simulink model "TorqueVect"  (R2022a)
settings: Solver=VariableStepAuto  StartTime=0.0  StopTime=300  RelTol=1e-3
PreLoadFcn:
  | run('Parameters\FSE_Parameters.m')
values from neighbouring files (symbols this model uses):
  Kd = 0;')    [open_carmaker_gui.m]
  Ki = 0    [open_carmaker_gui.m]
undefined symbols (not defined in the file or in its folder): BRegenEnabledButton, canChannel, CyalphaLookUp, efficiency, Fz_curve, Fz_scaling_long, gearR, izz, jw, kd, ki, Kp, kp, l_f, l_r, lambda, m, Mz_max, N, N_lat, N_long, P_max, pid_kd_lat, pid_kd_long, pid_ki_lat, pid_ki_long, pid_kp_lat, pid_kp_long, R_max, rw, steerR, T_i_max, TC_Decr_Gas, TC_Derivative, TC_Incr_Gas, TC_On, TC_Relay_Off, TC_Relay_On, tireCornerStiffness, Ts, TV_On, TV_Override, velocity_lookup, velocity_lookup_lat, y_ref, yrr_scaling
libraries: simulink x218, slpidlib x135, CarMaker4SL x73, TractionControlLibrary x13, canmsglib x9, canlib x8, TorqueVectoringLibrary x6, simulink_extras x4, PedalConversionLibrary x3, PowerControlLibrary x1
(part 9 of 26)

== system TorqueVect/CarMaker/IPG Vehicle/PowerTrain/PTControl Example/PTControl_ALL_Speedgoat/New TC/Reference Generator1 ==
  note: Modified slip ratio targets
  note: Vehicle velocity
  note: For throttle sign and Product:
      | If positive, normal reference
      | If negative (regen), similar reference but negative (negative target slip*times speed), this might need to change to account for regen limits
      | If 0, target zero
  x2 : Inport
  Front SR Target : Inport  Port=2
  Rear SR Target : Inport  Port=3
  Constant : Constant
  Product1 : Product
  Product2 : Product
  Switch : Switch  Criteria=u2 > Threshold  Threshold=1  SaturateOnIntegerOverflow=off  InputSameDT=off
  R1 : Outport
  L1 : Outport  Port=2
  R2 : Outport  Port=3
  L2 : Outport  Port=4
  wires:
  Front SR Target/1 -> Product1/1
  Product1/1 -> L1/1, R1/1
  Product2/1 -> L2/1, R2/1
  Rear SR Target/1 -> Product2/2
  Switch/1 -> Product2/1, Product1/2
  x2/1 -> Switch/1, Switch/2
  Constant/1 -> Switch/3

== system TorqueVect/CarMaker/IPG Vehicle/PowerTrain/PTControl Example/PTControl_ALL_Speedgoat/New TC/TC R1 ==
  modified slip ratio reference : Inport
  lim 1 : Inport  Port=2
  modified slip ratio measurement : Inport  Port=3
  P_TC : Inport  Port=4
  D_TC : Inport  Port=5
  enable_tc : Inport  Port=6
  PID Controller : slpidlib/PID Controller  Commented=on  Controller=PD  Form=Parallel  TimeDomain=Discrete-time  UseExternalTs=off  SampleTime=-1  IntegratorMethod=Forward Euler  FilterMethod=Forward Euler  ControllerParametersSource=external  P=125  I=1  UseKiTs=on  D=0  N=100  UseFilter=on  TunerSelectOption=Transfer Function Based (PID Tuner App)  InitialConditionSource=internal  InitialConditionForIntegrator=0  InitialConditionForFilter=0  DifferentiatorICPrevScaledInput=0  ExternalReset=none  TrackingMode=off  Kt=1  LimitOutput=on  SatLimitsSource=external  UpperSaturationLimit=inf  LowerSaturationLimit=-inf  LinearizeAsGain=on  AntiWindupMode=clamping  Kb=1  POutMin=[]  POutMax=[]  IOutMin=[]  IOutMax=[]  DOutMin=[]  DOutMax=[]  NOutMin=[]  NOutMax=[]  SumOutMin=[]  SumOutMax=[]  SaturationOutMin=[]  SaturationOutMax=[]  PParamMin=[]  PParamMax=[]  IParamMin=[]  IParamMax=[]  DParamMin=[]  DParamMax=[]  NParamMin=[]  NParamMax=[]  KbParamMin=[]  KbParamMax=[]  KtParamMin=[]  KtParamMax=[]  KbOutMin=[]  KbOutMax=[]  KtOutMin=[]  KtOutMax=[]  IntegratorOutMin=[]  IntegratorOutMax=[]  FilterOutMin=[]  FilterOutMax=[]  SumI1OutMin=[]  SumI1OutMax=[]  SumI2OutMin=[]  SumI2OutMax=[]  SumI3OutMin=[]  SumI3OutMax=[]  SumI4OutMin=[]  SumI4OutMax=[]  SumDOutMin=[]  SumDOutMax=[]  DifferentiatorOutMin=[]  DifferentiatorOutMax=[]  FilterDiffOutCoefMin=[]  FilterDiffOutCoefMax=[]  ReciprocalOutMin=[]  ReciprocalOutMax=[]  SumDenOutMin=[]  SumDenOutMax=[]  SumNumOutMin=[]  SumNumOutMax=[]  DivideOutMin=[]  DivideOutMax=[]  UdiffTsProdOutMin=[]  UdiffTsProdOutMax=[]  NTsProdOutMin=[]  NTsProdOutMax=[]  UintegralTsProdOutMin=[]  UintegralTsProdOutMax=[]  UngainTsProdOutMin=[]  UngainTsProdOutMax=[]  ClampingZeroOutDataTypeStr=Inherit: Inherit via back propagation  ClampingZeroOutMin=[]  ClampingZeroOutMax=[]  FilterDenConstantOutDataTypeStr=Inherit: Inherit via back propagation  FilterDenConstantOutMin=[]  FilterDenConstantOutMax=[]  PCopyOutDataTypeStr=Inherit: Inherit via back propagation  PCopyOutMin=[]  PCopyOutMax=[]  NCopyOutDataTypeStr=Inherit: Inherit via back propagation  NCopyOutMin=[]  NCopyOutMax=[]  IntegratorContinuousStateAttributes=''  IntegratorStateMustResolveToSignalObject=off  IntegratorRTWStateStorageClass=Auto  FilterContinuousStateAttributes=''  FilterStateMustResolveToSignalObject=off  FilterRTWStateStorageClass=Auto  ParallelPVariant=ExternalParameters  IdealPVariant=Disabled  IVariant=Disabled  DVariant=ExternalParameters  IntegratorVariant=Disabled  SatVariant=External  AWVariant=Disabled  PCopyVariant=Disabled  TRVariant=Disabled  FdbkBlocksVariant=Forward  IdealPFdbkVariant=Disabled  SatFdbkVariant=Disabled  DerivativeFilterVariant=ForwardEulerFilter  NVariant=ExternalParameters  NCopyVariant=Disabled  FilterICVariant=InternalICsFilter  IntegratorICVariant=Disabled  ExternalResetVariant=Disabled  TRSumVariant=Passthrough  SumFdbkVariant=Disabled  SumVariant=Sum_PD  TsampFilterVariant=InternalTs  TsampNgainVariant=Passthrough  TsampIntegralVariant=Disabled_SignalSpec  ExternalSaturationOutDataTypeStr=Inherit: Same as second input  aMode=0
  Sum1 : Sum  Inputs=|-+
  Sum2 : Sum  Commented=on  Inputs=|-+
  traction_controller : Subsystem
  Control Effort 1 : Outport
  wires:
  modified slip ratio reference/1 -> Sum1/1
  modified slip ratio measurement/1 -> Sum1/2
  lim 1/1 -> Sum2/2, traction_controller/1(max_torque)
  PID Controller/1 -> Sum2/1
  traction_controller/1(delta_torque) -> Control Effort 1/1
  enable_tc/1 -> traction_controller/3(enable_tc)
  Sum1/1 -> traction_controller/2(dslip)
  P_TC/1 -> traction_controller/4(Kp)
  D_TC/1 -> traction_controller/5(Kd)

== system TorqueVect/CarMaker/IPG Vehicle/PowerTrain/PTControl Example/PTControl_ALL_Speedgoat/New TC/TC R2 ==
  modified slip ratio reference : Inport
  lim 1 : Inport  Port=2
  modified slip ratio measurement : Inport  Port=3
  P_TC : Inport  Port=4
  D_TC : Inport  Port=5
  enable_tc : Inport  Port=6
  PID Controller : slpidlib/PID Controller  Commented=on  Controller=PD  Form=Parallel  TimeDomain=Discrete-time  UseExternalTs=off  SampleTime=-1  IntegratorMethod=Forward Euler  FilterMethod=Forward Euler  ControllerParametersSource=external  P=125  I=1  UseKiTs=on  D=0  N=100  UseFilter=on  TunerSelectOption=Transfer Function Based (PID Tuner App)  InitialConditionSource=internal  InitialConditionForIntegrator=0  InitialConditionForFilter=0  DifferentiatorICPrevScaledInput=0  ExternalReset=none  TrackingMode=off  Kt=1  LimitOutput=on  SatLimitsSource=external  UpperSaturationLimit=inf  LowerSaturationLimit=-inf  LinearizeAsGain=on  AntiWindupMode=clamping  Kb=1  POutMin=[]  POutMax=[]  IOutMin=[]  IOutMax=[]  DOutMin=[]  DOutMax=[]  NOutMin=[]  NOutMax=[]  SumOutMin=[]  SumOutMax=[]  SaturationOutMin=[]  SaturationOutMax=[]  PParamMin=[]  PParamMax=[]  IParamMin=[]  IParamMax=[]  DParamMin=[]  DParamMax=[]  NParamMin=[]  NParamMax=[]  KbParamMin=[]  KbParamMax=[]  KtParamMin=[]  KtParamMax=[]  KbOutMin=[]  KbOutMax=[]  KtOutMin=[]  KtOutMax=[]  IntegratorOutMin=[]  IntegratorOutMax=[]  FilterOutMin=[]  FilterOutMax=[]  SumI1OutMin=[]  SumI1OutMax=[]  SumI2OutMin=[]  SumI2OutMax=[]  SumI3OutMin=[]  SumI3OutMax=[]  SumI4OutMin=[]  SumI4OutMax=[]  SumDOutMin=[]  SumDOutMax=[]  DifferentiatorOutMin=[]  DifferentiatorOutMax=[]  FilterDiffOutCoefMin=[]  FilterDiffOutCoefMax=[]  ReciprocalOutMin=[]  ReciprocalOutMax=[]  SumDenOutMin=[]  SumDenOutMax=[]  SumNumOutMin=[]  SumNumOutMax=[]  DivideOutMin=[]  DivideOutMax=[]  UdiffTsProdOutMin=[]  UdiffTsProdOutMax=[]  NTsProdOutMin=[]  NTsProdOutMax=[]  UintegralTsProdOutMin=[]  UintegralTsProdOutMax=[]  UngainTsProdOutMin=[]  UngainTsProdOutMax=[]  ClampingZeroOutDataTypeStr=Inherit: Inherit via back propagation  ClampingZeroOutMin=[]  ClampingZeroOutMax=[]  FilterDenConstantOutDataTypeStr=Inherit: Inherit via back propagation  FilterDenConstantOutMin=[]  FilterDenConstantOutMax=[]  PCopyOutDataTypeStr=Inherit: Inherit via back propagation  PCopyOutMin=[]  PCopyOutMax=[]  NCopyOutDataTypeStr=Inherit: Inherit via back propagation  NCopyOutMin=[]  NCopyOutMax=[]  IntegratorContinuousStateAttributes=''  IntegratorStateMustResolveToSignalObject=off  IntegratorRTWStateStorageClass=Auto  FilterContinuousStateAttributes=''  FilterStateMustResolveToSignalObject=off  FilterRTWStateStorageClass=Auto  ParallelPVariant=ExternalParameters  IdealPVariant=Disabled  IVariant=Disabled  DVariant=ExternalParameters  IntegratorVariant=Disabled  SatVariant=External  AWVariant=Disabled  PCopyVariant=Disabled  TRVariant=Disabled  FdbkBlocksVariant=Forward  IdealPFdbkVariant=Disabled  SatFdbkVariant=Disabled  DerivativeFilterVariant=ForwardEulerFilter  NVariant=ExternalParameters  NCopyVariant=Disabled  FilterICVariant=InternalICsFilter  IntegratorICVariant=Disabled  ExternalResetVariant=Disabled  TRSumVariant=Passthrough  SumFdbkVariant=Disabled  SumVariant=Sum_PD  TsampFilterVariant=InternalTs  TsampNgainVariant=Passthrough  TsampIntegralVariant=Disabled_SignalSpec  ExternalSaturationOutDataTypeStr=Inherit: Same as second input  aMode=0
  Sum1 : Sum  Inputs=|-+
  Sum2 : Sum  Commented=on  Inputs=|-+
  traction_controller : Subsystem
  Control Effort 1 : Outport
  wires:
  modified slip ratio reference/1 -> Sum1/1
  modified slip ratio measurement/1 -> Sum1/2
  lim 1/1 -> Sum2/2, traction_controller/1(max_torque)
  PID Controller/1 -> Sum2/1
  traction_controller/1(delta_torque) -> Control Effort 1/1
  enable_tc/1 -> traction_controller/3(enable_tc)
  Sum1/1 -> traction_controller/2(dslip)
  P_TC/1 -> traction_controller/4(Kp)
  D_TC/1 -> traction_controller/5(Kd)

== system TorqueVect/CarMaker/IPG Vehicle/PowerTrain/PTControl Example/PTControl_ALL_Speedgoat/New TC/TC R3 ==
  modified slip ratio reference : Inport
  lim 1 : Inport  Port=2
  modified slip ratio measurement : Inport  Port=3
  P_TC : Inport  Port=4
  D_TC : Inport  Port=5
  enable_tc : Inport  Port=6
  PID Controller : slpidlib/PID Controller  Commented=on  Controller=PD  Form=Parallel  TimeDomain=Discrete-time  UseExternalTs=off  SampleTime=-1  IntegratorMethod=Forward Euler  FilterMethod=Forward Euler  ControllerParametersSource=external  P=125  I=1  UseKiTs=on  D=0  N=100  UseFilter=on  TunerSelectOption=Transfer Function Based (PID Tuner App)  InitialConditionSource=internal  InitialConditionForIntegrator=0  InitialConditionForFilter=0  DifferentiatorICPrevScaledInput=0  ExternalReset=none  TrackingMode=off  Kt=1  LimitOutput=on  SatLimitsSource=external  UpperSaturationLimit=inf  LowerSaturationLimit=-inf  LinearizeAsGain=on  AntiWindupMode=clamping  Kb=1  POutMin=[]  POutMax=[]  IOutMin=[]  IOutMax=[]  DOutMin=[]  DOutMax=[]  NOutMin=[]  NOutMax=[]  SumOutMin=[]  SumOutMax=[]  SaturationOutMin=[]  SaturationOutMax=[]  PParamMin=[]  PParamMax=[]  IParamMin=[]  IParamMax=[]  DParamMin=[]  DParamMax=[]  NParamMin=[]  NParamMax=[]  KbParamMin=[]  KbParamMax=[]  KtParamMin=[]  KtParamMax=[]  KbOutMin=[]  KbOutMax=[]  KtOutMin=[]  KtOutMax=[]  IntegratorOutMin=[]  IntegratorOutMax=[]  FilterOutMin=[]  FilterOutMax=[]  SumI1OutMin=[]  SumI1OutMax=[]  SumI2OutMin=[]  SumI2OutMax=[]  SumI3OutMin=[]  SumI3OutMax=[]  SumI4OutMin=[]  SumI4OutMax=[]  SumDOutMin=[]  SumDOutMax=[]  DifferentiatorOutMin=[]  DifferentiatorOutMax=[]  FilterDiffOutCoefMin=[]  FilterDiffOutCoefMax=[]  ReciprocalOutMin=[]  ReciprocalOutMax=[]  SumDenOutMin=[]  SumDenOutMax=[]  SumNumOutMin=[]  SumNumOutMax=[]  DivideOutMin=[]  DivideOutMax=[]  UdiffTsProdOutMin=[]  UdiffTsProdOutMax=[]  NTsProdOutMin=[]  NTsProdOutMax=[]  UintegralTsProdOutMin=[]  UintegralTsProdOutMax=[]  UngainTsProdOutMin=[]  UngainTsProdOutMax=[]  ClampingZeroOutDataTypeStr=Inherit: Inherit via back propagation  ClampingZeroOutMin=[]  ClampingZeroOutMax=[]  FilterDenConstantOutDataTypeStr=Inherit: Inherit via back propagation  FilterDenConstantOutMin=[]  FilterDenConstantOutMax=[]  PCopyOutDataTypeStr=Inherit: Inherit via back propagation  PCopyOutMin=[]  PCopyOutMax=[]  NCopyOutDataTypeStr=Inherit: Inherit via back propagation  NCopyOutMin=[]  NCopyOutMax=[]  IntegratorContinuousStateAttributes=''  IntegratorStateMustResolveToSignalObject=off  IntegratorRTWStateStorageClass=Auto  FilterContinuousStateAttributes=''  FilterStateMustResolveToSignalObject=off  FilterRTWStateStorageClass=Auto  ParallelPVariant=ExternalParameters  IdealPVariant=Disabled  IVariant=Disabled  DVariant=ExternalParameters  IntegratorVariant=Disabled  SatVariant=External  AWVariant=Disabled  PCopyVariant=Disabled  TRVariant=Disabled  FdbkBlocksVariant=Forward  IdealPFdbkVariant=Disabled  SatFdbkVariant=Disabled  DerivativeFilterVariant=ForwardEulerFilter  NVariant=ExternalParameters  NCopyVariant=Disabled  FilterICVariant=InternalICsFilter  IntegratorICVariant=Disabled  ExternalResetVariant=Disabled  TRSumVariant=Passthrough  SumFdbkVariant=Disabled  SumVariant=Sum_PD  TsampFilterVariant=InternalTs  TsampNgainVariant=Passthrough  TsampIntegralVariant=Disabled_SignalSpec  ExternalSaturationOutDataTypeStr=Inherit: Same as second input  aMode=0
  Sum1 : Sum  Inputs=|-+
  Sum2 : Sum  Commented=on  Inputs=|-+
  traction_controller : Subsystem
  Control Effort 1 : Outport
  wires:
  modified slip ratio reference/1 -> Sum1/1
  modified slip ratio measurement/1 -> Sum1/2
  lim 1/1 -> Sum2/2, traction_controller/1(max_torque)
  PID Controller/1 -> Sum2/1
  traction_controller/1(delta_torque) -> Control Effort 1/1
  enable_tc/1 -> traction_controller/3(enable_tc)
  Sum1/1 -> traction_controller/2(dslip)
  P_TC/1 -> traction_controller/4(Kp)
  D_TC/1 -> traction_controller/5(Kd)

== system TorqueVect/CarMaker/IPG Vehicle/PowerTrain/PTControl Example/PTControl_ALL_Speedgoat/New TC/TC R4 ==
  modified slip ratio reference : Inport
  lim 1 : Inport  Port=2
  modified slip ratio measurement : Inport  Port=3
  P_TC : Inport  Port=4
  D_TC : Inport  Port=5
  enable_tc : Inport  Port=6
  PID Controller : slpidlib/PID Controller  Commented=on  Controller=PD  Form=Parallel  TimeDomain=Discrete-time  UseExternalTs=off  SampleTime=-1  IntegratorMethod=Forward Euler  FilterMethod=Forward Euler  ControllerParametersSource=external  P=125  I=1  UseKiTs=on  D=0  N=100  UseFilter=on  TunerSelectOption=Transfer Function Based (PID Tuner App)  InitialConditionSource=internal  InitialConditionForIntegrator=0  InitialConditionForFilter=0  DifferentiatorICPrevScaledInput=0  ExternalReset=none  TrackingMode=off  Kt=1  LimitOutput=on  SatLimitsSource=external  UpperSaturationLimit=inf  LowerSaturationLimit=-inf  LinearizeAsGain=on  AntiWindupMode=clamping  Kb=1  POutMin=[]  POutMax=[]  IOutMin=[]  IOutMax=[]  DOutMin=[]  DOutMax=[]  NOutMin=[]  NOutMax=[]  SumOutMin=[]  SumOutMax=[]  SaturationOutMin=[]  SaturationOutMax=[]  PParamMin=[]  PParamMax=[]  IParamMin=[]  IParamMax=[]  DParamMin=[]  DParamMax=[]  NParamMin=[]  NParamMax=[]  KbParamMin=[]  KbParamMax=[]  KtParamMin=[]  KtParamMax=[]  KbOutMin=[]  KbOutMax=[]  KtOutMin=[]  KtOutMax=[]  IntegratorOutMin=[]  IntegratorOutMax=[]  FilterOutMin=[]  FilterOutMax=[]  SumI1OutMin=[]  SumI1OutMax=[]  SumI2OutMin=[]  SumI2OutMax=[]  SumI3OutMin=[]  SumI3OutMax=[]  SumI4OutMin=[]  SumI4OutMax=[]  SumDOutMin=[]  SumDOutMax=[]  DifferentiatorOutMin=[]  DifferentiatorOutMax=[]  FilterDiffOutCoefMin=[]  FilterDiffOutCoefMax=[]  ReciprocalOutMin=[]  ReciprocalOutMax=[]  SumDenOutMin=[]  SumDenOutMax=[]  SumNumOutMin=[]  SumNumOutMax=[]  DivideOutMin=[]  DivideOutMax=[]  UdiffTsProdOutMin=[]  UdiffTsProdOutMax=[]  NTsProdOutMin=[]  NTsProdOutMax=[]  UintegralTsProdOutMin=[]  UintegralTsProdOutMax=[]  UngainTsProdOutMin=[]  UngainTsProdOutMax=[]  ClampingZeroOutDataTypeStr=Inherit: Inherit via back propagation  ClampingZeroOutMin=[]  ClampingZeroOutMax=[]  FilterDenConstantOutDataTypeStr=Inherit: Inherit via back propagation  FilterDenConstantOutMin=[]  FilterDenConstantOutMax=[]  PCopyOutDataTypeStr=Inherit: Inherit via back propagation  PCopyOutMin=[]  PCopyOutMax=[]  NCopyOutDataTypeStr=Inherit: Inherit via back propagation  NCopyOutMin=[]  NCopyOutMax=[]  IntegratorContinuousStateAttributes=''  IntegratorStateMustResolveToSignalObject=off  IntegratorRTWStateStorageClass=Auto  FilterContinuousStateAttributes=''  FilterStateMustResolveToSignalObject=off  FilterRTWStateStorageClass=Auto  ParallelPVariant=ExternalParameters  IdealPVariant=Disabled  IVariant=Disabled  DVariant=ExternalParameters  IntegratorVariant=Disabled  SatVariant=External  AWVariant=Disabled  PCopyVariant=Disabled  TRVariant=Disabled  FdbkBlocksVariant=Forward  IdealPFdbkVariant=Disabled  SatFdbkVariant=Disabled  DerivativeFilterVariant=ForwardEulerFilter  NVariant=ExternalParameters  NCopyVariant=Disabled  FilterICVariant=InternalICsFilter  IntegratorICVariant=Disabled  ExternalResetVariant=Disabled  TRSumVariant=Passthrough  SumFdbkVariant=Disabled  SumVariant=Sum_PD  TsampFilterVariant=InternalTs  TsampNgainVariant=Passthrough  TsampIntegralVariant=Disabled_SignalSpec  ExternalSaturationOutDataTypeStr=Inherit: Same as second input  aMode=0
  Sum1 : Sum  Inputs=|-+
  Sum2 : Sum  Commented=on  Inputs=|-+
  traction_controller : Subsystem
  Control Effort 1 : Outport
  wires:
  modified slip ratio reference/1 -> Sum1/1
  modified slip ratio measurement/1 -> Sum1/2
  lim 1/1 -> Sum2/2, traction_controller/1(max_torque)
  PID Controller/1 -> Sum2/1
  traction_controller/1(delta_torque) -> Control Effort 1/1
  enable_tc/1 -> traction_controller/3(enable_tc)
  Sum1/1 -> traction_controller/2(dslip)
  P_TC/1 -> traction_controller/4(Kp)
  D_TC/1 -> traction_controller/5(Kd)

== system TorqueVect/CarMaker/IPG Vehicle/PowerTrain/PTControl Example/PTControl_ALL_Speedgoat/Subsystem/Subsystem ==
  Bus Creator : BusCreator  Inputs=5
  CAN Receive : canlib/CAN Receive  BlockHandle=92250.0002  Device=MathWorks Virtual 1 (Channel 1)  DeviceMenu=MathWorks Virtual 1 (Channel 1)  ObjConstructor=canChannel('MathWorks', 'Virtual 1', 1)  EnableStandardIDsFilter=off  StdIDsCombo=Allow all  StandardIDs=[111 211 311 411]  EnableExtendedIDsFilter=off  ExtIDsCombo=Allow all  ExtendedIDs=0  SampleTime=-1  MsgsPerTimestep=all  InternalFilterUpdateStatus=on  BusOutput=off
      settings: SourceProductBaseCode=VN
  CAN Unpack : canmsglib/CAN Unpack  MsgList=(none)  MsgName=Torques  MsgIDType=Standard (11-bit identifier)  MsgIdentifier=111  MsgLength=8  SignalInfo={ 'FL_Trq', '0', '16', 'LE', 'signed', 'Standard', '0', '1', '0', '-32768', '32767'; 'FR_Trq', '16', '16', 'LE', 'signed', 'Standard', '0', '1', '0', '-Inf', 'Inf'; 'RL_Trq', '32', '16', 'LE', 'signed', 'Standard', '0', '1', '0', '-Inf', 'Inf'; 'RR_Trq', '48', '16', 'LE', 'signed', 'Standard', '0', '1', '0', '-Inf', 'Inf' }  IDPort=off  TimestampPort=off  ErrorPort=off  RemotePort=off  LengthPort=off  StatusPort=off  ApplyMinMax=off
      settings: SourceProductBaseCode=ME,XP,VN
  CAN Unpack1 : canmsglib/CAN Unpack  MsgList=(none)  MsgName=Torques  MsgIDType=Standard (11-bit identifier)  MsgIdentifier=811  MsgLength=2  SignalInfo={ 'aSlip', '0', '16', 'LE', 'signed', 'Standard', '0', '1', '0', '-Inf', 'Inf' }  IDPort=off  TimestampPort=off  ErrorPort=off  RemotePort=off  LengthPort=off  StatusPort=off  ApplyMinMax=off
      settings: SourceProductBaseCode=ME,XP,VN
  Gain{,1..3} (4 alike) : Gain  Gain=1/98
  Gain4 : Gain  Gain=1/1000
  Terminator : Terminator
  Terminator1 : Terminator
  Trq : canmsglib/CAN Unpack  Commented=on  MsgList=(none)  MsgName=CAN Msg  MsgIDType=Standard (11-bit identifier)  MsgIdentifier=700  MsgLength=8  SignalInfo={ 'FL_Trq', '0', '16', 'LE', 'signed', 'Standard', '0', '1', '0', '-210', '210'; 'FR_Trq', '16', '16', 'LE', 'signed', 'Standard', '0', '1', '0', '-210', '210'; 'RL_Trq', '32', '16', 'LE', 'signed', 'Standard', '0', '1', '0', '-210', '210'; 'RR_Trq', '48', '16', 'LE', 'signed', 'Standard', '0', '1', '0', '-210', '210' }  IDPort=off  TimestampPort=off  ErrorPort=off  RemotePort=off  LengthPort=off  StatusPort=off  ApplyMinMax=off
      settings: SourceProductBaseCode=ME,XP,VN
  Out1 : Outport
  Out2 : Outport  Port=2
  Out3 : Outport  Port=3
  Out4 : Outport  Port=4
  wires:
  CAN Unpack/2 -> Gain1/1
  CAN Unpack/1 -> Gain/1
  CAN Unpack/3 -> Gain2/1
  CAN Unpack/4 -> Gain3/1
  CAN Receive/1 -> Terminator/1
  Gain/1 -> Bus Creator/1, Out1/1  "fl_trq"
  Gain1/1 -> Bus Creator/2, Out2/1  "fr_trq"
  Gain2/1 -> Bus Creator/3, Out3/1  "rl_trq"
  Gain3/1 -> Bus Creator/4, Out4/1  "rr_trq"
  Bus Creator/1 -> Terminator1/1  "rec_can"
  CAN Receive/2 -> CAN Unpack1/1, CAN Unpack/1
  CAN Unpack1/1 -> Gain4/1
  Gain4/1 -> Bus Creator/5

== system TorqueVect/CarMaker/IPG Vehicle/PowerTrain/PTControl Example/PTControl_PC_MFE/New TC/Reference Generator1 ==
  note: Modified slip ratio targets
  note: Vehicle velocity
  note: For throttle sign and Product:
      | If positive, normal reference
      | If negative (regen), similar reference but negative (negative target slip*times speed), this might need to change to account for regen limits
      | If 0, target zero
  x2 : Inport
  Front SR Target : Inport  Port=2
  Rear SR Target : Inport  Port=3
  Constant : Constant
  Product1 : Product
  Product2 : Product
  Switch : Switch  Criteria=u2 > Threshold  Threshold=1  SaturateOnIntegerOverflow=off  InputSameDT=off
  R1 : Outport
  L1 : Outport  Port=2
  R2 : Outport  Port=3
  L2 : Outport  Port=4
  wires:
  Front SR Target/1 -> Product1/1
  Product1/1 -> L1/1, R1/1
  Product2/1 -> L2/1, R2/1
  Rear SR Target/1 -> Product2/2
  Switch/1 -> Product2/1, Product1/2
  x2/1 -> Switch/1, Switch/2
  Constant/1 -> Switch/3

== system TorqueVect/CarMaker/IPG Vehicle/PowerTrain/PTControl Example/PTControl_PC_MFE/New TC/TC R1 ==
  modified slip ratio reference : Inport
  lim 1 : Inport  Port=2
  modified slip ratio measurement : Inport  Port=3
  P_TC : Inport  Port=4
  D_TC : Inport  Port=5
  enable_tc : Inport  Port=6
  PID Controller : slpidlib/PID Controller  Commented=on  Controller=PD  Form=Parallel  TimeDomain=Discrete-time  UseExternalTs=off  SampleTime=-1  IntegratorMethod=Forward Euler  FilterMethod=Forward Euler  ControllerParametersSource=external  P=125  I=1  UseKiTs=on  D=0  N=100  UseFilter=on  TunerSelectOption=Transfer Function Based (PID Tuner App)  InitialConditionSource=internal  InitialConditionForIntegrator=0  InitialConditionForFilter=0  DifferentiatorICPrevScaledInput=0  ExternalReset=none  TrackingMode=off  Kt=1  LimitOutput=on  SatLimitsSource=external  UpperSaturationLimit=inf  LowerSaturationLimit=-inf  LinearizeAsGain=on  AntiWindupMode=clamping  Kb=1  POutMin=[]  POutMax=[]  IOutMin=[]  IOutMax=[]  DOutMin=[]  DOutMax=[]  NOutMin=[]  NOutMax=[]  SumOutMin=[]  SumOutMax=[]  SaturationOutMin=[]  SaturationOutMax=[]  PParamMin=[]  PParamMax=[]  IParamMin=[]  IParamMax=[]  DParamMin=[]  DParamMax=[]  NParamMin=[]  NParamMax=[]  KbParamMin=[]  KbParamMax=[]  KtParamMin=[]  KtParamMax=[]  KbOutMin=[]  KbOutMax=[]  KtOutMin=[]  KtOutMax=[]  IntegratorOutMin=[]  IntegratorOutMax=[]  FilterOutMin=[]  FilterOutMax=[]  SumI1OutMin=[]  SumI1OutMax=[]  SumI2OutMin=[]  SumI2OutMax=[]  SumI3OutMin=[]  SumI3OutMax=[]  SumI4OutMin=[]  SumI4OutMax=[]  SumDOutMin=[]  SumDOutMax=[]  DifferentiatorOutMin=[]  DifferentiatorOutMax=[]  FilterDiffOutCoefMin=[]  FilterDiffOutCoefMax=[]  ReciprocalOutMin=[]  ReciprocalOutMax=[]  SumDenOutMin=[]  SumDenOutMax=[]  SumNumOutMin=[]  SumNumOutMax=[]  DivideOutMin=[]  DivideOutMax=[]  UdiffTsProdOutMin=[]  UdiffTsProdOutMax=[]  NTsProdOutMin=[]  NTsProdOutMax=[]  UintegralTsProdOutMin=[]  UintegralTsProdOutMax=[]  UngainTsProdOutMin=[]  UngainTsProdOutMax=[]  ClampingZeroOutDataTypeStr=Inherit: Inherit via back propagation  ClampingZeroOutMin=[]  ClampingZeroOutMax=[]  FilterDenConstantOutDataTypeStr=Inherit: Inherit via back propagation  FilterDenConstantOutMin=[]  FilterDenConstantOutMax=[]  PCopyOutDataTypeStr=Inherit: Inherit via back propagation  PCopyOutMin=[]  PCopyOutMax=[]  NCopyOutDataTypeStr=Inherit: Inherit via back propagation  NCopyOutMin=[]  NCopyOutMax=[]  IntegratorContinuousStateAttributes=''  IntegratorStateMustResolveToSignalObject=off  IntegratorRTWStateStorageClass=Auto  FilterContinuousStateAttributes=''  FilterStateMustResolveToSignalObject=off  FilterRTWStateStorageClass=Auto  ParallelPVariant=ExternalParameters  IdealPVariant=Disabled  IVariant=Disabled  DVariant=ExternalParameters  IntegratorVariant=Disabled  SatVariant=External  AWVariant=Disabled  PCopyVariant=Disabled  TRVariant=Disabled  FdbkBlocksVariant=Forward  IdealPFdbkVariant=Disabled  SatFdbkVariant=Disabled  DerivativeFilterVariant=ForwardEulerFilter  NVariant=ExternalParameters  NCopyVariant=Disabled  FilterICVariant=InternalICsFilter  IntegratorICVariant=Disabled  ExternalResetVariant=Disabled  TRSumVariant=Passthrough  SumFdbkVariant=Disabled  SumVariant=Sum_PD  TsampFilterVariant=InternalTs  TsampNgainVariant=Passthrough  TsampIntegralVariant=Disabled_SignalSpec  ExternalSaturationOutDataTypeStr=Inherit: Same as second input  aMode=0
  Sum1 : Sum  Inputs=|-+
  Sum2 : Sum  Commented=on  Inputs=|-+
  traction_controller : Subsystem
  Control Effort 1 : Outport
  wires:
  modified slip ratio reference/1 -> Sum1/1
  modified slip ratio measurement/1 -> Sum1/2
  lim 1/1 -> Sum2/2, traction_controller/1(max_torque)
  PID Controller/1 -> Sum2/1
  traction_controller/1(delta_torque) -> Control Effort 1/1
  enable_tc/1 -> traction_controller/3(enable_tc)
  Sum1/1 -> traction_controller/2(dslip)
  P_TC/1 -> traction_controller/4(Kp)
  D_TC/1 -> traction_controller/5(Kd)

== system TorqueVect/CarMaker/IPG Vehicle/PowerTrain/PTControl Example/PTControl_PC_MFE/New TC/TC R2 ==
  modified slip ratio reference : Inport
  lim 1 : Inport  Port=2
  modified slip ratio measurement : Inport  Port=3
  P_TC : Inport  Port=4
  D_TC : Inport  Port=5
  enable_tc : Inport  Port=6
  PID Controller : slpidlib/PID Controller  Commented=on  Controller=PD  Form=Parallel  TimeDomain=Discrete-time  UseExternalTs=off  SampleTime=-1  IntegratorMethod=Forward Euler  FilterMethod=Forward Euler  ControllerParametersSource=external  P=125  I=1  UseKiTs=on  D=0  N=100  UseFilter=on  TunerSelectOption=Transfer Function Based (PID Tuner App)  InitialConditionSource=internal  InitialConditionForIntegrator=0  InitialConditionForFilter=0  DifferentiatorICPrevScaledInput=0  ExternalReset=none  TrackingMode=off  Kt=1  LimitOutput=on  SatLimitsSource=external  UpperSaturationLimit=inf  LowerSaturationLimit=-inf  LinearizeAsGain=on  AntiWindupMode=clamping  Kb=1  POutMin=[]  POutMax=[]  IOutMin=[]  IOutMax=[]  DOutMin=[]  DOutMax=[]  NOutMin=[]  NOutMax=[]  SumOutMin=[]  SumOutMax=[]  SaturationOutMin=[]  SaturationOutMax=[]  PParamMin=[]  PParamMax=[]  IParamMin=[]  IParamMax=[]  DParamMin=[]  DParamMax=[]  NParamMin=[]  NParamMax=[]  KbParamMin=[]  KbParamMax=[]  KtParamMin=[]  KtParamMax=[]  KbOutMin=[]  KbOutMax=[]  KtOutMin=[]  KtOutMax=[]  IntegratorOutMin=[]  IntegratorOutMax=[]  FilterOutMin=[]  FilterOutMax=[]  SumI1OutMin=[]  SumI1OutMax=[]  SumI2OutMin=[]  SumI2OutMax=[]  SumI3OutMin=[]  SumI3OutMax=[]  SumI4OutMin=[]  SumI4OutMax=[]  SumDOutMin=[]  SumDOutMax=[]  DifferentiatorOutMin=[]  DifferentiatorOutMax=[]  FilterDiffOutCoefMin=[]  FilterDiffOutCoefMax=[]  ReciprocalOutMin=[]  ReciprocalOutMax=[]  SumDenOutMin=[]  SumDenOutMax=[]  SumNumOutMin=[]  SumNumOutMax=[]  DivideOutMin=[]  DivideOutMax=[]  UdiffTsProdOutMin=[]  UdiffTsProdOutMax=[]  NTsProdOutMin=[]  NTsProdOutMax=[]  UintegralTsProdOutMin=[]  UintegralTsProdOutMax=[]  UngainTsProdOutMin=[]  UngainTsProdOutMax=[]  ClampingZeroOutDataTypeStr=Inherit: Inherit via back propagation  ClampingZeroOutMin=[]  ClampingZeroOutMax=[]  FilterDenConstantOutDataTypeStr=Inherit: Inherit via back propagation  FilterDenConstantOutMin=[]  FilterDenConstantOutMax=[]  PCopyOutDataTypeStr=Inherit: Inherit via back propagation  PCopyOutMin=[]  PCopyOutMax=[]  NCopyOutDataTypeStr=Inherit: Inherit via back propagation  NCopyOutMin=[]  NCopyOutMax=[]  IntegratorContinuousStateAttributes=''  IntegratorStateMustResolveToSignalObject=off  IntegratorRTWStateStorageClass=Auto  FilterContinuousStateAttributes=''  FilterStateMustResolveToSignalObject=off  FilterRTWStateStorageClass=Auto  ParallelPVariant=ExternalParameters  IdealPVariant=Disabled  IVariant=Disabled  DVariant=ExternalParameters  IntegratorVariant=Disabled  SatVariant=External  AWVariant=Disabled  PCopyVariant=Disabled  TRVariant=Disabled  FdbkBlocksVariant=Forward  IdealPFdbkVariant=Disabled  SatFdbkVariant=Disabled  DerivativeFilterVariant=ForwardEulerFilter  NVariant=ExternalParameters  NCopyVariant=Disabled  FilterICVariant=InternalICsFilter  IntegratorICVariant=Disabled  ExternalResetVariant=Disabled  TRSumVariant=Passthrough  SumFdbkVariant=Disabled  SumVariant=Sum_PD  TsampFilterVariant=InternalTs  TsampNgainVariant=Passthrough  TsampIntegralVariant=Disabled_SignalSpec  ExternalSaturationOutDataTypeStr=Inherit: Same as second input  aMode=0
  Sum1 : Sum  Inputs=|-+
  Sum2 : Sum  Commented=on  Inputs=|-+
  traction_controller : Subsystem
  Control Effort 1 : Outport
  wires:
  modified slip ratio reference/1 -> Sum1/1
  modified slip ratio measurement/1 -> Sum1/2
  lim 1/1 -> Sum2/2, traction_controller/1(max_torque)
  PID Controller/1 -> Sum2/1
  traction_controller/1(delta_torque) -> Control Effort 1/1
  enable_tc/1 -> traction_controller/3(enable_tc)
  Sum1/1 -> traction_controller/2(dslip)
  P_TC/1 -> traction_controller/4(Kp)
  D_TC/1 -> traction_controller/5(Kd)

== system TorqueVect/CarMaker/IPG Vehicle/PowerTrain/PTControl Example/PTControl_PC_MFE/New TC/TC R3 ==
  modified slip ratio reference : Inport
  lim 1 : Inport  Port=2
  modified slip ratio measurement : Inport  Port=3
  P_TC : Inport  Port=4
  D_TC : Inport  Port=5
  enable_tc : Inport  Port=6
  PID Controller : slpidlib/PID Controller  Commented=on  Controller=PD  Form=Parallel  TimeDomain=Discrete-time  UseExternalTs=off  SampleTime=-1  IntegratorMethod=Forward Euler  FilterMethod=Forward Euler  ControllerParametersSource=external  P=125  I=1  UseKiTs=on  D=0  N=100  UseFilter=on  TunerSelectOption=Transfer Function Based (PID Tuner App)  InitialConditionSource=internal  InitialConditionForIntegrator=0  InitialConditionForFilter=0  DifferentiatorICPrevScaledInput=0  ExternalReset=none  TrackingMode=off  Kt=1  LimitOutput=on  SatLimitsSource=external  UpperSaturationLimit=inf  LowerSaturationLimit=-inf  LinearizeAsGain=on  AntiWindupMode=clamping  Kb=1  POutMin=[]  POutMax=[]  IOutMin=[]  IOutMax=[]  DOutMin=[]  DOutMax=[]  NOutMin=[]  NOutMax=[]  SumOutMin=[]  SumOutMax=[]  SaturationOutMin=[]  SaturationOutMax=[]  PParamMin=[]  PParamMax=[]  IParamMin=[]  IParamMax=[]  DParamMin=[]  DParamMax=[]  NParamMin=[]  NParamMax=[]  KbParamMin=[]  KbParamMax=[]  KtParamMin=[]  KtParamMax=[]  KbOutMin=[]  KbOutMax=[]  KtOutMin=[]  KtOutMax=[]  IntegratorOutMin=[]  IntegratorOutMax=[]  FilterOutMin=[]  FilterOutMax=[]  SumI1OutMin=[]  SumI1OutMax=[]  SumI2OutMin=[]  SumI2OutMax=[]  SumI3OutMin=[]  SumI3OutMax=[]  SumI4OutMin=[]  SumI4OutMax=[]  SumDOutMin=[]  SumDOutMax=[]  DifferentiatorOutMin=[]  DifferentiatorOutMax=[]  FilterDiffOutCoefMin=[]  FilterDiffOutCoefMax=[]  ReciprocalOutMin=[]  ReciprocalOutMax=[]  SumDenOutMin=[]  SumDenOutMax=[]  SumNumOutMin=[]  SumNumOutMax=[]  DivideOutMin=[]  DivideOutMax=[]  UdiffTsProdOutMin=[]  UdiffTsProdOutMax=[]  NTsProdOutMin=[]  NTsProdOutMax=[]  UintegralTsProdOutMin=[]  UintegralTsProdOutMax=[]  UngainTsProdOutMin=[]  UngainTsProdOutMax=[]  ClampingZeroOutDataTypeStr=Inherit: Inherit via back propagation  ClampingZeroOutMin=[]  ClampingZeroOutMax=[]  FilterDenConstantOutDataTypeStr=Inherit: Inherit via back propagation  FilterDenConstantOutMin=[]  FilterDenConstantOutMax=[]  PCopyOutDataTypeStr=Inherit: Inherit via back propagation  PCopyOutMin=[]  PCopyOutMax=[]  NCopyOutDataTypeStr=Inherit: Inherit via back propagation  NCopyOutMin=[]  NCopyOutMax=[]  IntegratorContinuousStateAttributes=''  IntegratorStateMustResolveToSignalObject=off  IntegratorRTWStateStorageClass=Auto  FilterContinuousStateAttributes=''  FilterStateMustResolveToSignalObject=off  FilterRTWStateStorageClass=Auto  ParallelPVariant=ExternalParameters  IdealPVariant=Disabled  IVariant=Disabled  DVariant=ExternalParameters  IntegratorVariant=Disabled  SatVariant=External  AWVariant=Disabled  PCopyVariant=Disabled  TRVariant=Disabled  FdbkBlocksVariant=Forward  IdealPFdbkVariant=Disabled  SatFdbkVariant=Disabled  DerivativeFilterVariant=ForwardEulerFilter  NVariant=ExternalParameters  NCopyVariant=Disabled  FilterICVariant=InternalICsFilter  IntegratorICVariant=Disabled  ExternalResetVariant=Disabled  TRSumVariant=Passthrough  SumFdbkVariant=Disabled  SumVariant=Sum_PD  TsampFilterVariant=InternalTs  TsampNgainVariant=Passthrough  TsampIntegralVariant=Disabled_SignalSpec  ExternalSaturationOutDataTypeStr=Inherit: Same as second input  aMode=0
  Sum1 : Sum  Inputs=|-+
  Sum2 : Sum  Commented=on  Inputs=|-+
  traction_controller : Subsystem
  Control Effort 1 : Outport
  wires:
  modified slip ratio reference/1 -> Sum1/1
  modified slip ratio measurement/1 -> Sum1/2
  lim 1/1 -> Sum2/2, traction_controller/1(max_torque)
  PID Controller/1 -> Sum2/1
  traction_controller/1(delta_torque) -> Control Effort 1/1
  enable_tc/1 -> traction_controller/3(enable_tc)
  Sum1/1 -> traction_controller/2(dslip)
  P_TC/1 -> traction_controller/4(Kp)
  D_TC/1 -> traction_controller/5(Kd)

== system TorqueVect/CarMaker/IPG Vehicle/PowerTrain/PTControl Example/PTControl_PC_MFE/New TC/TC R4 ==
  modified slip ratio reference : Inport
  lim 1 : Inport  Port=2
  modified slip ratio measurement : Inport  Port=3
  P_TC : Inport  Port=4
  D_TC : Inport  Port=5
  enable_tc : Inport  Port=6
  PID Controller : slpidlib/PID Controller  Commented=on  Controller=PD  Form=Parallel  TimeDomain=Discrete-time  UseExternalTs=off  SampleTime=-1  IntegratorMethod=Forward Euler  FilterMethod=Forward Euler  ControllerParametersSource=external  P=125  I=1  UseKiTs=on  D=0  N=100  UseFilter=on  TunerSelectOption=Transfer Function Based (PID Tuner App)  InitialConditionSource=internal  InitialConditionForIntegrator=0  InitialConditionForFilter=0  DifferentiatorICPrevScaledInput=0  ExternalReset=none  TrackingMode=off  Kt=1  LimitOutput=on  SatLimitsSource=external  UpperSaturationLimit=inf  LowerSaturationLimit=-inf  LinearizeAsGain=on  AntiWindupMode=clamping  Kb=1  POutMin=[]  POutMax=[]  IOutMin=[]  IOutMax=[]  DOutMin=[]  DOutMax=[]  NOutMin=[]  NOutMax=[]  SumOutMin=[]  SumOutMax=[]  SaturationOutMin=[]  SaturationOutMax=[]  PParamMin=[]  PParamMax=[]  IParamMin=[]  IParamMax=[]  DParamMin=[]  DParamMax=[]  NParamMin=[]  NParamMax=[]  KbParamMin=[]  KbParamMax=[]  KtParamMin=[]  KtParamMax=[]  KbOutMin=[]  KbOutMax=[]  KtOutMin=[]  KtOutMax=[]  IntegratorOutMin=[]  IntegratorOutMax=[]  FilterOutMin=[]  FilterOutMax=[]  SumI1OutMin=[]  SumI1OutMax=[]  SumI2OutMin=[]  SumI2OutMax=[]  SumI3OutMin=[]  SumI3OutMax=[]  SumI4OutMin=[]  SumI4OutMax=[]  SumDOutMin=[]  SumDOutMax=[]  DifferentiatorOutMin=[]  DifferentiatorOutMax=[]  FilterDiffOutCoefMin=[]  FilterDiffOutCoefMax=[]  ReciprocalOutMin=[]  ReciprocalOutMax=[]  SumDenOutMin=[]  SumDenOutMax=[]  SumNumOutMin=[]  SumNumOutMax=[]  DivideOutMin=[]  DivideOutMax=[]  UdiffTsProdOutMin=[]  UdiffTsProdOutMax=[]  NTsProdOutMin=[]  NTsProdOutMax=[]  UintegralTsProdOutMin=[]  UintegralTsProdOutMax=[]  UngainTsProdOutMin=[]  UngainTsProdOutMax=[]  ClampingZeroOutDataTypeStr=Inherit: Inherit via back propagation  ClampingZeroOutMin=[]  ClampingZeroOutMax=[]  FilterDenConstantOutDataTypeStr=Inherit: Inherit via back propagation  FilterDenConstantOutMin=[]  FilterDenConstantOutMax=[]  PCopyOutDataTypeStr=Inherit: Inherit via back propagation  PCopyOutMin=[]  PCopyOutMax=[]  NCopyOutDataTypeStr=Inherit: Inherit via back propagation  NCopyOutMin=[]  NCopyOutMax=[]  IntegratorContinuousStateAttributes=''  IntegratorStateMustResolveToSignalObject=off  IntegratorRTWStateStorageClass=Auto  FilterContinuousStateAttributes=''  FilterStateMustResolveToSignalObject=off  FilterRTWStateStorageClass=Auto  ParallelPVariant=ExternalParameters  IdealPVariant=Disabled  IVariant=Disabled  DVariant=ExternalParameters  IntegratorVariant=Disabled  SatVariant=External  AWVariant=Disabled  PCopyVariant=Disabled  TRVariant=Disabled  FdbkBlocksVariant=Forward  IdealPFdbkVariant=Disabled  SatFdbkVariant=Disabled  DerivativeFilterVariant=ForwardEulerFilter  NVariant=ExternalParameters  NCopyVariant=Disabled  FilterICVariant=InternalICsFilter  IntegratorICVariant=Disabled  ExternalResetVariant=Disabled  TRSumVariant=Passthrough  SumFdbkVariant=Disabled  SumVariant=Sum_PD  TsampFilterVariant=InternalTs  TsampNgainVariant=Passthrough  TsampIntegralVariant=Disabled_SignalSpec  ExternalSaturationOutDataTypeStr=Inherit: Same as second input  aMode=0
  Sum1 : Sum  Inputs=|-+
  Sum2 : Sum  Commented=on  Inputs=|-+
  traction_controller : Subsystem
  Control Effort 1 : Outport
  wires:
  modified slip ratio reference/1 -> Sum1/1
  modified slip ratio measurement/1 -> Sum1/2
  lim 1/1 -> Sum2/2, traction_controller/1(max_torque)
  PID Controller/1 -> Sum2/1
  traction_controller/1(delta_torque) -> Control Effort 1/1
  enable_tc/1 -> traction_controller/3(enable_tc)
  Sum1/1 -> traction_controller/2(dslip)
  P_TC/1 -> traction_controller/4(Kp)
  D_TC/1 -> traction_controller/5(Kd)

== system TorqueVect/CarMaker/IPG Vehicle/PowerTrain/PTControl Example/PTControl_PC_MFE/Subsystem/PowerControl ==
  MMotorFL : Inport  OutMin=-42  OutMax=42  Unit=N*m  PortDimensions=1
      settings: AttributesFormatString=[%<OutMin>, %<OutMax>] %<Unit>
  MMotorFR : Inport  Port=2  OutMin=-42  OutMax=42  Unit=N*m  PortDimensions=1
      settings: AttributesFormatString=[%<OutMin>, %<OutMax>] %<Unit>
  MMotorRL : Inport  Port=3  OutMin=-42  OutMax=42  Unit=N*m  PortDimensions=1
      settings: AttributesFormatString=[%<OutMin>, %<OutMax>] %<Unit>
  MMotorRR : Inport  Port=4  OutMin=-42  OutMax=42  Unit=N*m  PortDimensions=1
      settings: AttributesFormatString=[%<OutMin>, %<OutMax>] %<Unit>
  nMotorFL : Inport  Port=5  OutMin=-3000  OutMax=3000  Unit=rad/s  PortDimensions=1
      settings: AttributesFormatString=[%<OutMin>, %<OutMax>] %<Unit>
  nMotorFR : Inport  Port=6  OutMin=-3000  OutMax=3000  Unit=rad/s  PortDimensions=1
      settings: AttributesFormatString=[%<OutMin>, %<OutMax>] %<Unit>
  nMotorRL : Inport  Port=7  OutMin=-3000  OutMax=3000  Unit=rad/s  PortDimensions=1
      settings: AttributesFormatString=[%<OutMin>, %<OutMax>] %<Unit>
  nMotorRR : Inport  Port=8  OutMin=-3000  OutMax=3000  Unit=rad/s  PortDimensions=1
      settings: AttributesFormatString=[%<OutMin>, %<OutMax>] %<Unit>
  PMeasured : Inport  Port=9  OutMin=-250000  OutMax=250000  Unit=W  PortDimensions=1
      settings: AttributesFormatString=[%<OutMin>, %<OutMax>] %<Unit>
  BMeasuredEnable : Inport  Port=10  OutMin=0  OutMax=1  PortDimensions=1
      settings: AttributesFormatString=[%<OutMin> / %<OutMax>]
  BRegenEnable : Inport  Port=11  OutMin=0  OutMax=1  PortDimensions=1
      settings: AttributesFormatString=[%<OutMin> / %<OutMax>]
  rSplitF : Inport  Port=12  OutMin=0  OutMax=1  PortDimensions=1
      settings: AttributesFormatString=[%<OutMin>, %<OutMax>]
  rThrottlePedal : Inport  Port=13  OutMin=0  OutMax=1  PortDimensions=1
      settings: AttributesFormatString=[%<OutMin>, %<OutMax>]
  rThrottle : Inport  Port=14  OutMin=-1  OutMax=1  PortDimensions=1
      settings: AttributesFormatString=[%<OutMin>, %<OutMax>]
  PRegenLimit : Inport  Port=15  OutMin=0  OutMax=80000  Unit=W  PortDimensions=1
      settings: AttributesFormatString=[%<OutMin>, %<OutMax>] %<Unit>
  PLimit : Inport  Port=16  OutMin=0  OutMax=80000  Unit=W  PortDimensions=1
      settings: AttributesFormatString=[%<OutMin>, %<OutMax>] %<Unit>
  FF_PC : Inport  Port=17
  FF_RC : Inport  Port=18
  P_PC : Inport  Port=19
  D_PC : Inport  Port=20
  PID : Subsystem
  PowerError : Subsystem
  PowerSplitF/R : Subsystem
  RegenError : Subsystem
  ResetPID_PC : Subsystem
  TotalPower : Subsystem
  WheelTorqueOut : Subsystem
  MReductionMotorFL : Outport  OutMin=0  OutMax=21  Unit=N*m  PortDimensions=1
      settings: AttributesFormatString=[%<OutMin>, %<OutMax>] %<Unit>
  MReductionMotorFR : Outport  Port=2  OutMin=0  OutMax=21  Unit=N*m  PortDimensions=1
      settings: AttributesFormatString=[%<OutMin>, %<OutMax>] %<Unit>
  MReductionMotorRL : Outport  Port=3  OutMin=0  OutMax=21  Unit=N*m  PortDimensions=1
      settings: AttributesFormatString=[%<OutMin>, %<OutMax>] %<Unit>
  MReductionMotorRR : Outport  Port=4  OutMin=0  OutMax=21  Unit=N*m  PortDimensions=1
      settings: AttributesFormatString=[%<OutMin>, %<OutMax>] %<Unit>
  wires:
  WheelTorqueOut/4(MReductionMotorRR) -> MReductionMotorRR/1
  WheelTorqueOut/3(MReductionMotorRL) -> MReductionMotorRL/1
  WheelTorqueOut/2(MReductionMotorFR) -> MReductionMotorFR/1
  WheelTorqueOut/1(MReductionMotorFL) -> MReductionMotorFL/1
  D_PC/1 -> PID/4(D_PC)
  P_PC/1 -> PID/3(P_PC)
  FF_RC/1 -> RegenError/2(FF_RC)
  FF_PC/1 -> PowerError/2(FF_PC)
  PLimit/1 -> PowerError/3(PLimit)
  PRegenLimit/1 -> RegenError/3(PRegenLimit)
  rThrottle/1 -> RegenError/4(rThrottle)
  rSplitF/1 -> PowerSplitF/R/2(rSplitF)
  BRegenEnable/1 -> ResetPID_PC/2(BRegenEnabled)
  rThrottlePedal/1 -> ResetPID_PC/1(rThrottlePedal)
  [nMotorRR] -> WheelTorqueOut/6(nMotorRR)
  [nMotorRL] -> WheelTorqueOut/5(nMotorRL)
  [nMotorFR] -> WheelTorqueOut/4(nMotorFR)
  [nMotorFL] -> WheelTorqueOut/3(nMotorFL)
  MMotorRR/1 -> TotalPower/7(MMotorRR)
  MMotorRL/1 -> TotalPower/5(MMotorRL)
  MMotorFR/1 -> TotalPower/3(MMotorFR)
  BMeasuredEnable/1 -> TotalPower/10(BMeasuredEnable)
  PMeasured/1 -> TotalPower/9(PMeasured)
  [nMotorRR] -> TotalPower/8(nMotorRR)
  [nMotorRL] -> TotalPower/6(nMotorRL)
  [nMotorFR] -> TotalPower/4(nMotorFR)
  [nMotorFL] -> TotalPower/2(nMotorFL)
  nMotorRR/1 -> [nMotorRR]
  nMotorRL/1 -> [nMotorRL]
  nMotorFR/1 -> [nMotorFR]
  nMotorFL/1 -> [nMotorFL]
  MMotorFL/1 -> TotalPower/1(MMotorFL)
  PowerSplitF/R/2(PReductionR) -> WheelTorqueOut/2(PReductionR)
  PowerSplitF/R/1(PReductionF) -> WheelTorqueOut/1(PReductionF)
  PID/1(PReductionTotal) -> PowerSplitF/R/1(PReductionTotal)
  ResetPID_PC/1(ResetPID_PC) -> PID/5(ResetPID_PC)
  RegenError/1(PRegenError) -> PID/2(PRegenError)
  PowerError/1(PError) -> PID/1(PError)
  TotalPower/2(PTotal) -> RegenError/1(PTotal)
  TotalPower/1(PPositiveTotal) -> PowerError/1(PPositiveTotal)

== system TorqueVect/CarMaker/IPG Vehicle/PowerTrain/PTControl Example/PTControl_PC_TC_MFE/New TC/Reference Generator1 ==
  note: Modified slip ratio targets
  note: Vehicle velocity
  note: For throttle sign and Product:
      | If positive, normal reference
      | If negative (regen), similar reference but negative (negative target slip*times speed), this might need to change to account for regen limits
      | If 0, target zero
  x2 : Inport
  Front SR Target : Inport  Port=2
  Rear SR Target : Inport  Port=3
  Constant : Constant
  Product1 : Product
  Product2 : Product
  Switch : Switch  Criteria=u2 > Threshold  Threshold=1  SaturateOnIntegerOverflow=off  InputSameDT=off
  R1 : Outport
  L1 : Outport  Port=2
  R2 : Outport  Port=3
  L2 : Outport  Port=4
  wires:
  Front SR Target/1 -> Product1/1
  Product1/1 -> L1/1, R1/1
  Product2/1 -> L2/1, R2/1
  Rear SR Target/1 -> Product2/2
  Switch/1 -> Product2/1, Product1/2
  x2/1 -> Switch/1, Switch/2
  Constant/1 -> Switch/3

== system TorqueVect/CarMaker/IPG Vehicle/PowerTrain/PTControl Example/PTControl_PC_TC_MFE/New TC/TC R1 ==
  modified slip ratio reference : Inport
  lim 1 : Inport  Port=2
  modified slip ratio measurement : Inport  Port=3
  P_TC : Inport  Port=4
  D_TC : Inport  Port=5
  enable_tc : Inport  Port=6
  PID Controller : slpidlib/PID Controller  Commented=on  Controller=PD  Form=Parallel  TimeDomain=Discrete-time  UseExternalTs=off  SampleTime=-1  IntegratorMethod=Forward Euler  FilterMethod=Forward Euler  ControllerParametersSource=external  P=125  I=1  UseKiTs=on  D=0  N=100  UseFilter=on  TunerSelectOption=Transfer Function Based (PID Tuner App)  InitialConditionSource=internal  InitialConditionForIntegrator=0  InitialConditionForFilter=0  DifferentiatorICPrevScaledInput=0  ExternalReset=none  TrackingMode=off  Kt=1  LimitOutput=on  SatLimitsSource=external  UpperSaturationLimit=inf  LowerSaturationLimit=-inf  LinearizeAsGain=on  AntiWindupMode=clamping  Kb=1  POutMin=[]  POutMax=[]  IOutMin=[]  IOutMax=[]  DOutMin=[]  DOutMax=[]  NOutMin=[]  NOutMax=[]  SumOutMin=[]  SumOutMax=[]  SaturationOutMin=[]  SaturationOutMax=[]  PParamMin=[]  PParamMax=[]  IParamMin=[]  IParamMax=[]  DParamMin=[]  DParamMax=[]  NParamMin=[]  NParamMax=[]  KbParamMin=[]  KbParamMax=[]  KtParamMin=[]  KtParamMax=[]  KbOutMin=[]  KbOutMax=[]  KtOutMin=[]  KtOutMax=[]  IntegratorOutMin=[]  IntegratorOutMax=[]  FilterOutMin=[]  FilterOutMax=[]  SumI1OutMin=[]  SumI1OutMax=[]  SumI2OutMin=[]  SumI2OutMax=[]  SumI3OutMin=[]  SumI3OutMax=[]  SumI4OutMin=[]  SumI4OutMax=[]  SumDOutMin=[]  SumDOutMax=[]  DifferentiatorOutMin=[]  DifferentiatorOutMax=[]  FilterDiffOutCoefMin=[]  FilterDiffOutCoefMax=[]  ReciprocalOutMin=[]  ReciprocalOutMax=[]  SumDenOutMin=[]  SumDenOutMax=[]  SumNumOutMin=[]  SumNumOutMax=[]  DivideOutMin=[]  DivideOutMax=[]  UdiffTsProdOutMin=[]  UdiffTsProdOutMax=[]  NTsProdOutMin=[]  NTsProdOutMax=[]  UintegralTsProdOutMin=[]  UintegralTsProdOutMax=[]  UngainTsProdOutMin=[]  UngainTsProdOutMax=[]  ClampingZeroOutDataTypeStr=Inherit: Inherit via back propagation  ClampingZeroOutMin=[]  ClampingZeroOutMax=[]  FilterDenConstantOutDataTypeStr=Inherit: Inherit via back propagation  FilterDenConstantOutMin=[]  FilterDenConstantOutMax=[]  PCopyOutDataTypeStr=Inherit: Inherit via back propagation  PCopyOutMin=[]  PCopyOutMax=[]  NCopyOutDataTypeStr=Inherit: Inherit via back propagation  NCopyOutMin=[]  NCopyOutMax=[]  IntegratorContinuousStateAttributes=''  IntegratorStateMustResolveToSignalObject=off  IntegratorRTWStateStorageClass=Auto  FilterContinuousStateAttributes=''  FilterStateMustResolveToSignalObject=off  FilterRTWStateStorageClass=Auto  ParallelPVariant=ExternalParameters  IdealPVariant=Disabled  IVariant=Disabled  DVariant=ExternalParameters  IntegratorVariant=Disabled  SatVariant=External  AWVariant=Disabled  PCopyVariant=Disabled  TRVariant=Disabled  FdbkBlocksVariant=Forward  IdealPFdbkVariant=Disabled  SatFdbkVariant=Disabled  DerivativeFilterVariant=ForwardEulerFilter  NVariant=ExternalParameters  NCopyVariant=Disabled  FilterICVariant=InternalICsFilter  IntegratorICVariant=Disabled  ExternalResetVariant=Disabled  TRSumVariant=Passthrough  SumFdbkVariant=Disabled  SumVariant=Sum_PD  TsampFilterVariant=InternalTs  TsampNgainVariant=Passthrough  TsampIntegralVariant=Disabled_SignalSpec  ExternalSaturationOutDataTypeStr=Inherit: Same as second input  aMode=0
  Sum1 : Sum  Inputs=|-+
  Sum2 : Sum  Commented=on  Inputs=|-+
  traction_controller : Subsystem
  Control Effort 1 : Outport
  wires:
  modified slip ratio reference/1 -> Sum1/1
  modified slip ratio measurement/1 -> Sum1/2
  lim 1/1 -> Sum2/2, traction_controller/1(max_torque)
  PID Controller/1 -> Sum2/1
  traction_controller/1(delta_torque) -> Control Effort 1/1
  enable_tc/1 -> traction_controller/3(enable_tc)
  Sum1/1 -> traction_controller/2(dslip)
  P_TC/1 -> traction_controller/4(Kp)
  D_TC/1 -> traction_controller/5(Kd)
